simulink model "EdgeDetectionAndOverlayHDLExample"  (R2018b)
settings: Solver=FixedStepDiscrete  StartTime=0.0  StopTime=1650*750*10  RelTol=1e-3
PreLoadFcn:
  | thresholdValue = 7;
  | alpha = 0.8;
undefined symbols (not defined in the file): gray
libraries: visionhdlio x2, visionanalysis x1, simulink x1, visionstatistics x1, hdlsllib x1, simulink_need_slupdate x1, visionhdlanalysis x1, dspvision x1
CloseFcn:
  | clear thresholdValue alpha;
settings Model: DataTypeOverride=Off  ModifiedByFormat=The MathWorks Inc.  SimulationMode=accelerator  Creator=The MathWorks, Inc.  LastModifiedBy=The MathWorks Inc.
settings DataIOCC: LimitDataPoints=on  SaveFormat=Array  SaveOutput=off  SaveTime=off
settings OptimizationCC: BlockReduction=off  ConditionallyExecuteInputs=off  DefaultParameterBehavior=Inlined  LifeSpan=inf
settings DebuggingCC: AlgebraicLoopMsg=error  SolverPrmCheckMsg=warning  SingleTaskRateTransMsg=error  ParameterPrecisionLossMsg=none  AllowSymbolicDim=off  SFUnexpectedBacktrackingDiag=warning  SFNoUnconditionalDefaultTransitionDiag=warning  IntegerSaturationMsg=none
settings HardwareCC: ProdBitPerPointer=32  ProdBitPerSizeT=32  ProdBitPerPtrDiffT=32  ProdLargestAtomicFloat=None  ProdIntDivRoundTo=Undefined  ProdEndianess=Unspecified  ProdWordSize=32  ProdHWDeviceType=ASIC/FPGA->ASIC/FPGA  ProdEqTarget=off
settings ModelReferenceCC: PropagateSignalLabelsOutOfModel=off
settings SFSimCC: SimUseLocalCustomCode=off
settings RTWCC: RTWUseLocalCustomCode=off
settings CodeAppCC: StateflowObjectComments=on
settings GRTTargetCC: TargetLangStandard=C89/C90 (ANSI)  GeneratePreprocessorConditionals=Disable all
settings ConfigComp: CovMetricSettings=dw  CovHtmlReporting=on  CovSaveCumulativeToWorkspaceVar=on  CovSaveSingleToWorkspaceVar=on  CovExternalEMLEnable=off  CovSFcnEnable=off

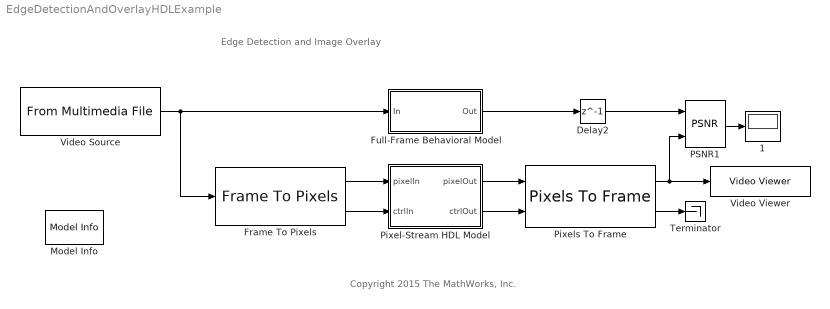
== system EdgeDetectionAndOverlayHDLExample ==
  note: Edge Detection and Image Overlay
  note: Copyright 2015 The MathWorks, Inc.
  " 1" : Display
  Delay2 : Delay  DelayLength=1  InitialCondition=0
  Frame To Pixels : visionhdlio/Frame To Pixels  NumComponents=1  VideoFormat=720p  ActivePixelsPerLine=800  ActiveVideoLines=600  TotalPixelsPerLine=1056  TotalVideoLines=628  StartingActiveLine=23  FrontPorch=40  SampleTime=0
      settings: SourceProductName=Vision HDL Toolbox  SourceProductBaseCode=VT
  Full-Frame Behavioral Model : Subsystem
  Model Info : simulink/Model-Wide Utilities/Model Info  Frame=on  DisplayStringWithTags=Info  HorizontalTextAlignment=Center  LeftAlignmentValue=0.5
  PSNR1 : visionstatistics/PSNR
      settings: SourceProductName=Computer Vision System Toolbox  SourceProductBaseCode=VP
  Pixel-Stream HDL Model : Subsystem  TreatAsAtomicUnit=on
  Pixels To Frame : visionhdlio/Pixels To Frame  NumComponents=1  VideoFormat=720p  ActivePixelsPerLine=800  ActiveVideoLines=600  TotalPixelsPerLine=1056  TotalVideoLines=628
      settings: SourceProductName=Vision HDL Toolbox  SourceProductBaseCode=VT
  Terminator : Terminator
  Video Source : dspvision/From Multimedia File  inputFilename=D:\ImageLabs\lab9\matlab\720p_BigBuckBunny.mp4  loop=on  numPlays=inf  outputStreams=Video only  videoDataType=uint8  audioDataType=int16  inheritSampleTime=off  userDefinedSampleTime=1650*750  noAudioOutput=off  isIntensityVideo=off  fourcc=Intensity  colorVideoFormat=One multidimensional signal  outputEOF=off  dataOrg=Column-major  audioFrameSize=1024  computeAudioFrameSize=off  outSamplingMode=Sample based
      settings: SourceProductBaseCode=VP
  Video Viewer : VideoViewer  colormapValue=gray(256)  FigPos=[1118 956 528 398]
  wires:
  Pixels To Frame/2 -> Terminator/1
  Video Source/1 -> Frame To Pixels/1, Full-Frame Behavioral Model/1(In)
  Full-Frame Behavioral Model/1(Out) -> Delay2/1
  PSNR1/1 -> " 1"/1
  Delay2/1 -> PSNR1/1
  Pixels To Frame/1 -> Video Viewer/1, PSNR1/2
  Frame To Pixels/1 -> Pixel-Stream HDL Model/1(pixelIn)
  Frame To Pixels/2 -> Pixel-Stream HDL Model/2(ctrlIn)
  Pixel-Stream HDL Model/1(pixelOut) -> Pixels To Frame/1
  Pixel-Stream HDL Model/2(ctrlOut) -> Pixels To Frame/2

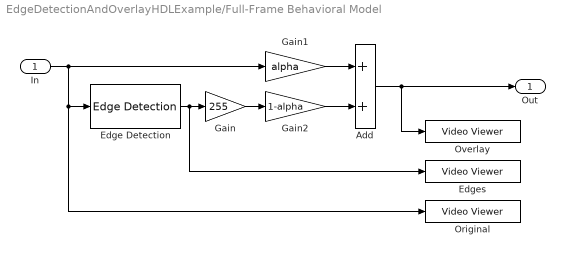
== system EdgeDetectionAndOverlayHDLExample/Full-Frame Behavioral Model ==
  In : Inport
  Add : Sum  OutDataTypeStr=uint8  SaturateOnIntegerOverflow=on
  Edge Detection : visionanalysis/Edge Detection  method=Sobel  outputType=Binary image  userDefinedThreshold=on  thresholdSource=Specify via dialog  threshold=thresholdValue  thresholdTuning=4  edgeThinning=off  threshold_canny=[0.25 0.60]  autoPercent=70  sigma=1  roundingMode=Floor  overflowMode=on  prodOutputMode=Binary point scaling  prodOutputWordLength=32  prodOutputFracLength=18  prodOutputSlope=2^-8  accumSlope=2^-8  outputSlope=2^-4
      settings: SourceProductName=Computer Vision System Toolbox  SourceProductBaseCode=VP
  Edges : VideoViewer  colormapValue=gray(256)  FigPos=[450 525 467 285]
  Gain : Gain  Gain=255  OutDataTypeStr=uint8
  Gain1 : Gain  Gain=alpha  OutDataTypeStr=uint8
  Gain2 : Gain  Gain=1-alpha  OutDataTypeStr=uint8
  Original : VideoViewer  colormapValue=gray(256)  FigPos=[454 525 459 285]
  Overlay : VideoViewer  colormapValue=gray(256)  FigPos=[450 525 466 285]
  Out : Outport
  wires:
  Gain/1 -> Gain2/1
  Gain1/1 -> Add/1
  Gain2/1 -> Add/2
  Edge Detection/1 -> Gain/1, Edges/1
  In/1 -> Original/1, Edge Detection/1, Gain1/1
  Add/1 -> Overlay/1, Out/1

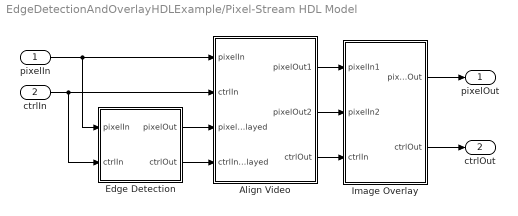
== system EdgeDetectionAndOverlayHDLExample/Pixel-Stream HDL Model ==
  pixelIn : Inport
  ctrlIn : Inport  Port=2
  Align Video : Subsystem
  Edge Detection : Subsystem
  Image Overlay : Subsystem
  pixelOut : Outport
  ctrlOut : Outport  Port=2
  wires:
  ctrlIn/1 -> Align Video/2(ctrlIn), Edge Detection/2(ctrlIn)
  pixelIn/1 -> Edge Detection/1(pixelIn), Align Video/1(pixelIn)
  Align Video/1(pixelOut1) -> Image Overlay/1(pixelIn1)
  Align Video/2(pixelOut2) -> Image Overlay/2(pixelIn2)
  Align Video/3(ctrlOut) -> Image Overlay/3(ctrlIn)
  Image Overlay/1(pixelOut) -> pixelOut/1
  Image Overlay/2(ctrlOut) -> ctrlOut/1
  Edge Detection/1(pixelOut) -> Align Video/3(pixelInDelayed)
  Edge Detection/2(ctrlOut) -> Align Video/4(ctrlInDelayed)

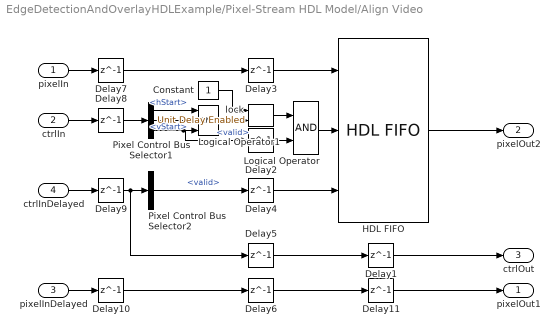
== system EdgeDetectionAndOverlayHDLExample/Pixel-Stream HDL Model/Align Video ==
  pixelIn : Inport
  ctrlIn : Inport  Port=2
  pixelInDelayed : Inport  Port=3
  ctrlInDelayed : Inport  Port=4
  Constant : Constant  OutDataTypeStr=boolean  SampleTime=1
  Delay{1..11} (11 alike) : Delay  DelayLength=1  InitialCondition=0
  HDL FIFO : hdlsllib/HDL RAMs/HDL FIFO  fifo_size=2048  ratio=1  push_msg=Warning  pop_msg=Warning  show_empty=off  show_full=off  show_num=off
      settings: SourceProductName=HDL Coder  SourceProductBaseCode=HD
  Logical Operator : Logic  AllPortsSameDT=off  OutDataTypeStr=boolean
  Logical Operator1 : Logic  Inputs=3  AllPortsSameDT=off  OutDataTypeStr=boolean
  Pixel Control Bus Selector1 : BusSelector  OutputSignals=hStart,vStart,valid
  Pixel Control Bus Selector2 : BusSelector  OutputSignals=valid
  lock : simulink_need_slupdate/Unit Delay Enabled  vinit=false  tsamp=1
      settings: SourceProductName=Simulink  SourceProductBaseCode=SL
  pixelOut1 : Outport
  pixelOut2 : Outport  Port=2
  ctrlOut : Outport  Port=3
  wires:
  pixelInDelayed/1 -> Delay10/1
  HDL FIFO/1 -> pixelOut2/1
  ctrlInDelayed/1 -> Delay9/1
  ctrlIn/1 -> Delay8/1
  pixelIn/1 -> Delay7/1
  Delay6/1 -> Delay11/1
  Delay5/1 -> Delay1/1
  Delay4/1 -> HDL FIFO/3
  Delay3/1 -> HDL FIFO/1
  Pixel Control Bus Selector1/3 -> Delay2/1, Logical Operator1/3  "<valid>"
  Delay2/1 -> Logical Operator/2
  Constant/1 -> lock/1
  lock/1 -> Logical Operator/1
  Logical Operator/1 -> HDL FIFO/2
  Pixel Control Bus Selector2/1 -> Delay4/1  "<valid>"
  Delay7/1 -> Delay3/1
  Delay10/1 -> Delay6/1
  Delay8/1 -> Pixel Control Bus Selector1/1
  Delay9/1 -> Pixel Control Bus Selector2/1, Delay5/1
  Logical Operator1/1 -> lock/2
  Pixel Control Bus Selector1/2 -> Logical Operator1/2  "<vStart>"
  Pixel Control Bus Selector1/1 -> Logical Operator1/1  "<hStart>"
  Delay1/1 -> ctrlOut/1
  Delay11/1 -> pixelOut1/1

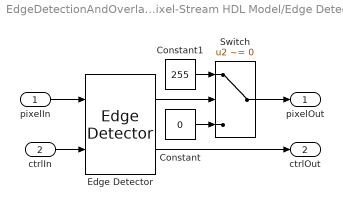
== system EdgeDetectionAndOverlayHDLExample/Pixel-Stream HDL Model/Edge Detection ==
  pixelIn : Inport
  ctrlIn : Inport  Port=2
  Constant : Constant  Value=0  OutDataTypeStr=uint8  SampleTime=1
  Constant1 : Constant  Value=255  OutDataTypeStr=uint8  SampleTime=1
  Edge Detector : visionhdlanalysis/Edge Detector  Method=Sobel  BinaryImageOutputPort=on  GradientComponentOutputPorts=off  ThresholdSource=Property  Threshold=thresholdValue  LineBufferSize=2048  SimulateUsing=Code generation  roundingMode=Floor  overflowMode=on  GradientMin=[]  GradientMax=[]
      settings: SourceProductName=Vision HDL Toolbox  SourceProductBaseCode=VT
  Switch : Switch  Criteria=u2 ~= 0
  pixelOut : Outport
  ctrlOut : Outport  Port=2
  wires:
  Constant1/1 -> Switch/1
  Edge Detector/1 -> Switch/2
  Constant/1 -> Switch/3
  Switch/1 -> pixelOut/1
  Edge Detector/2 -> ctrlOut/1
  ctrlIn/1 -> Edge Detector/2
  pixelIn/1 -> Edge Detector/1

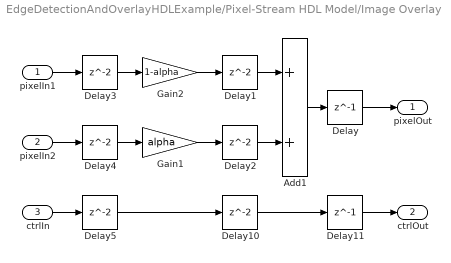
== system EdgeDetectionAndOverlayHDLExample/Pixel-Stream HDL Model/Image Overlay ==
  pixelIn1 : Inport
  pixelIn2 : Inport  Port=2
  ctrlIn : Inport  Port=3
  Add1 : Sum  OutDataTypeStr=uint8  SaturateOnIntegerOverflow=on
  Delay : Delay  DelayLength=1  InitialCondition=0
  Delay{1..5,10} (6 alike) : Delay  InitialCondition=0
  Delay11 : Delay  DelayLength=1  InitialCondition=0
  Gain1 : Gain  Gain=alpha  OutDataTypeStr=uint8
  Gain2 : Gain  Gain=1-alpha  OutDataTypeStr=uint8
  pixelOut : Outport
  ctrlOut : Outport  Port=2
  wires:
  Delay11/1 -> ctrlOut/1
  pixelIn1/1 -> Delay3/1
  ctrlIn/1 -> Delay5/1
  Gain1/1 -> Delay2/1
  Delay3/1 -> Gain2/1
  Delay/1 -> pixelOut/1
  Gain2/1 -> Delay1/1
  Delay1/1 -> Add1/1
  Delay10/1 -> Delay11/1
  Delay4/1 -> Gain1/1
  Add1/1 -> Delay/1
  Delay2/1 -> Add1/2
  Delay5/1 -> Delay10/1
  pixelIn2/1 -> Delay4/1
